simulink model "dualConversionSuperheterodyneKuBandReceiver"  (R2021b)
settings: Solver=VariableStepAuto  StartTime=0.0  StopTime=10.0  RelTol=1e-3
undefined symbols (not defined in the file): fdesignblkfcn, gcbh
libraries: dsparch4 x6, dspsrcs4 x4
settings Model: Creator=Zireael  LastModifiedBy=Zireael

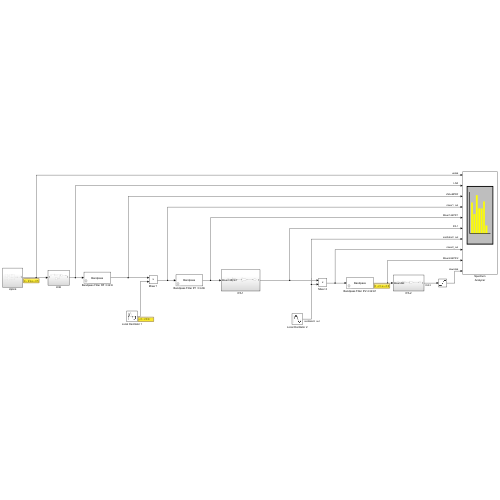
[thumbnail: Simulink's stored preview of the top-level diagram]
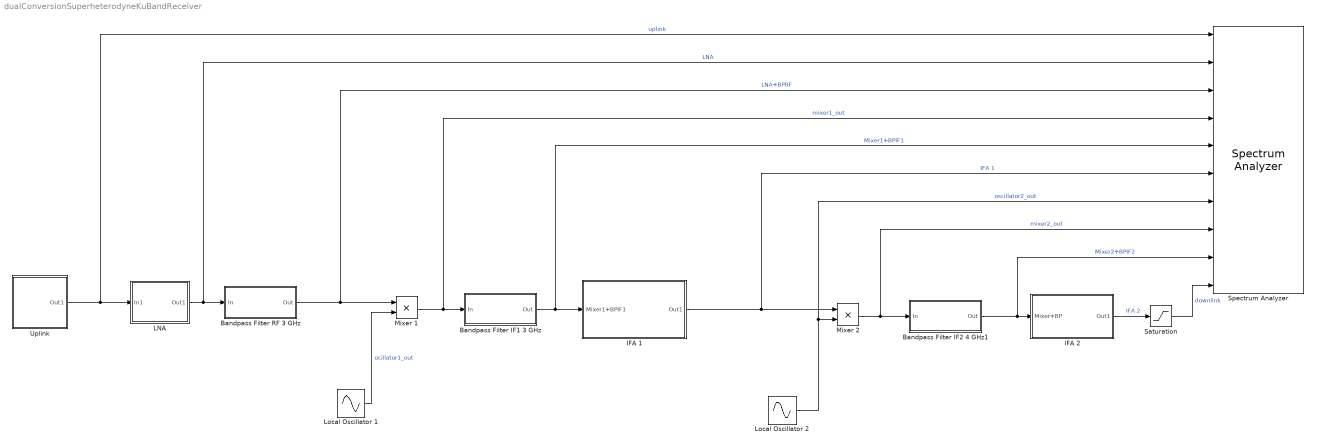
== system dualConversionSuperheterodyneKuBandReceiver ==
  Bandpass Filter IF1 3 GHz : Subsystem  DialogController=fdesignblkfcn  InitFcn=fdesignblkfcn(gcbh, {'InitFcn'});  mask(Bandpass Filter){}
      mask help: Design a bandpass filter
      settings: CopyFcn=fdesignblkfcn(gcbh, {'CopyFcn'});
      mask Help: helpview(mapfilelocation('dsp'), 'dspbandpassfilter');
      mask Display: disp('Bandpass');
  Bandpass Filter IF2 4 GHz1 : Subsystem  DialogController=fdesignblkfcn  InitFcn=fdesignblkfcn(gcbh, {'InitFcn'});  mask(Bandpass Filter){}
      mask help: Design a bandpass filter
      settings: CopyFcn=fdesignblkfcn(gcbh, {'CopyFcn'});
      mask Help: helpview(mapfilelocation('dsp'), 'dspbandpassfilter');
      mask Display: disp('Bandpass');
  Bandpass Filter RF 3 GHz : Subsystem  DialogController=fdesignblkfcn  InitFcn=fdesignblkfcn(gcbh, {'InitFcn'});  mask(Bandpass Filter){}
      mask help: Design a bandpass filter
      settings: CopyFcn=fdesignblkfcn(gcbh, {'CopyFcn'});
      mask Help: helpview(mapfilelocation('dsp'), 'dspbandpassfilter');
      mask Display: disp('Bandpass');
  IFA 1 : Subsystem
  IFA 2 : Subsystem
  LNA : Subsystem
  Local Oscillator 1 : Sin  Frequency=2*pi*2225e6  SampleTime=1/(50e9)
  Local Oscillator 2 : Sin  Frequency=2*pi*2225e6  SampleTime=1/(50e9)
  Mixer 1 : Product
  Mixer 2 : Product
  Saturation : Saturate  UpperLimit=0.9e4  LowerLimit=-0.9e4
  Spectrum Analyzer : SpectrumAnalyzer  NumInputPorts=10
  Uplink : Subsystem
  wires:
  Local Oscillator 1/1 -> Mixer 1/2  "ocillator1_out"
  Uplink/1(Out1) -> Spectrum Analyzer/1, LNA/1(In1)  "uplink"
  Bandpass Filter RF 3 GHz/1(Out) -> Spectrum Analyzer/3, Mixer 1/1  "LNA+BPRF"
  LNA/1(Out1) -> Spectrum Analyzer/2, Bandpass Filter RF 3 GHz/1(In)  "LNA"
  Mixer 1/1 -> Spectrum Analyzer/4, Bandpass Filter IF1 3 GHz/1(In)  "mixer1_out"
  Bandpass Filter IF1 3 GHz/1(Out) -> Spectrum Analyzer/5, IFA 1/1(Mixer1+BPIF1)  "Mixer1+BPIF1"
  Local Oscillator 2/1 -> Mixer 2/2, Spectrum Analyzer/7  "oscillator2_out"
  Mixer 2/1 -> Spectrum Analyzer/8, Bandpass Filter IF2 4 GHz1/1(In)  "mixer2_out"
  Bandpass Filter IF2 4 GHz1/1(Out) -> Spectrum Analyzer/9, IFA 2/1(Mixer+BP)  "Mixer2+BPIF2"
  IFA 1/1(Out1) -> Spectrum Analyzer/6, Mixer 2/1  "IFA 1"
  IFA 2/1(Out1) -> Saturation/1  "IFA 2"
  Saturation/1 -> Spectrum Analyzer/10  "downlink"

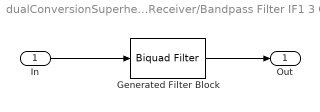
== system dualConversionSuperheterodyneKuBandReceiver/Bandpass Filter IF1 3 GHz ==
  In : Inport
  Generated Filter Block : dsparch4/Biquad Filter  Tag=BlockMethodSubSystem  FilterSource=Dialog parameters  CoeffSource=Specify via dialog  FilterObject=BQF  IIRFiltStruct=Direct form II  BiQuadCoeffs=[0.0449395006068324179 0 -0.0449395006068324179 1 0.405266255527262198 0.993681559777048418;0.0151701499365588764 0 -0.0151701499365588764 1 0.317251182402427279 0.993629226472784288;0.0102846537000260332 0 -0.0102846537000260332 1 0.370702484346910832 0.991152828113709083;0.0156527649221751067 0 -0.0156527649221751067 1 0.351249848252692232 0.991136685128483963;0.0620781828063547217 0 -0.0620781828063547217 1 0.423582164672003603 0.998601688644412899;0.00934586574907354285 0 -0.00934586574907354285 1 0.300377452446864479 0.998585448434978429;0.0223874419851657382 0 -0.0223874419851657382 1 0.389303276704848988 0.992030706822551345;0.0130129978737727608 0 -0.0130129978737727608 1 0.332830940728660596 0.991988419043733027;0.059531840912397431 0 -0.059531840912397431 1 0.417068161267263871 0.995944293101420075;0.511470005384135895 0 -0.511470005384135895 1 0.306057042862860063 0.995901877379559486]  ScaleValues=[0.00618861187356475363;1;1;1;1;1;1;1;1;1;1]  IC=0  ICnum=0  ICden=0  a0Flag=Warning  optimizeScaleValues=off  ScaleValueMode=Specify via input port (g)  InputProcessing=Columns as channels (frame based)  roundingMode=Floor  overflowMode=off  scaleValueFracLength=14  denProdOutputFracLength=30  denAccumFracLength=30  secondMemoryFracLength=15
  Out : Outport  VectorParamsAs1DForOutWhenUnconnected=off
  wires:
  In/1 -> Generated Filter Block/1
  Generated Filter Block/1 -> Out/1

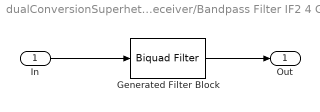
== system dualConversionSuperheterodyneKuBandReceiver/Bandpass Filter IF2 4 GHz1 ==
  In : Inport
  Generated Filter Block : dsparch4/Biquad Filter  Tag=BlockMethodSubSystem  FilterSource=Dialog parameters  CoeffSource=Specify via dialog  FilterObject=BQF  IIRFiltStruct=Direct form II  BiQuadCoeffs=[0.0449395006068324179 0 -0.0449395006068324179 1 0.405266255527262198 0.993681559777048418;0.0151701499365588764 0 -0.0151701499365588764 1 0.317251182402427279 0.993629226472784288;0.0102846537000260332 0 -0.0102846537000260332 1 0.370702484346910832 0.991152828113709083;0.0156527649221751067 0 -0.0156527649221751067 1 0.351249848252692232 0.991136685128483963;0.0620781828063547217 0 -0.0620781828063547217 1 0.423582164672003603 0.998601688644412899;0.00934586574907354285 0 -0.00934586574907354285 1 0.300377452446864479 0.998585448434978429;0.0223874419851657382 0 -0.0223874419851657382 1 0.389303276704848988 0.992030706822551345;0.0130129978737727608 0 -0.0130129978737727608 1 0.332830940728660596 0.991988419043733027;0.059531840912397431 0 -0.059531840912397431 1 0.417068161267263871 0.995944293101420075;0.511470005384135895 0 -0.511470005384135895 1 0.306057042862860063 0.995901877379559486]  ScaleValues=[0.00618861187356475363;1;1;1;1;1;1;1;1;1;1]  IC=0  ICnum=0  ICden=0  a0Flag=Warning  optimizeScaleValues=off  ScaleValueMode=Specify via input port (g)  InputProcessing=Columns as channels (frame based)  roundingMode=Floor  overflowMode=off  scaleValueFracLength=14  denProdOutputFracLength=30  denAccumFracLength=30  secondMemoryFracLength=15
  Out : Outport  VectorParamsAs1DForOutWhenUnconnected=off
  wires:
  In/1 -> Generated Filter Block/1
  Generated Filter Block/1 -> Out/1

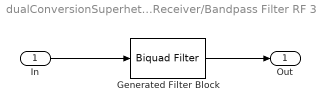
== system dualConversionSuperheterodyneKuBandReceiver/Bandpass Filter RF 3 GHz ==
  In : Inport
  Generated Filter Block : dsparch4/Biquad Filter  Tag=BlockMethodSubSystem  FilterSource=Dialog parameters  CoeffSource=Specify via dialog  FilterObject=BQF  IIRFiltStruct=Direct form II  BiQuadCoeffs=[0.0449015005721064217 0 -0.0449015005721064217 1 0.460304770997229384 0.993685734471094873;0.0151718610592496122 0 -0.0151718610592496122 1 0.372780342872187143 0.993625052016134158;0.010292301404864557 0 -0.010292301404864557 1 0.425888978774519256 0.991154115861604401;0.0155960047074426896 0 -0.0155960047074426896 1 0.406544551045089853 0.991135397403234641;0.0623098100146096748 0 -0.0623098100146096748 1 0.478631344122104563 0.998602984094145718;0.0093415546403119807 0 -0.0093415546403119807 1 0.356116647279347776 0.998584153007991748;0.0223945390284251249 0 -0.0223945390284251249 1 0.444400611296275394 0.992034080197356283;0.0130197808043754238 0 -0.0130197808043754238 1 0.388242637402923141 0.991985045824199996;0.0594862648562931723 0 -0.0594862648562931723 1 0.472088444940327034 0.995947676595487108;0.514535971971806561 0 -0.514535971971806561 1 0.36169744229138806 0.995898494041079996]  ScaleValues=[0.00615350492122296311;1;1;1;1;1;1;1;1;1;1]  IC=0  ICnum=0  ICden=0  a0Flag=Warning  optimizeScaleValues=off  ScaleValueMode=Specify via input port (g)  InputProcessing=Columns as channels (frame based)  roundingMode=Floor  overflowMode=off  scaleValueFracLength=14  denProdOutputFracLength=30  denAccumFracLength=30  secondMemoryFracLength=15
  Out : Outport  VectorParamsAs1DForOutWhenUnconnected=off
  wires:
  In/1 -> Generated Filter Block/1
  Generated Filter Block/1 -> Out/1

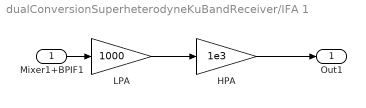
== system dualConversionSuperheterodyneKuBandReceiver/IFA 1 ==
  Mixer1+BPIF1 : Inport
  HPA : Gain  Gain=1e3
  LPA : Gain  Gain=1000
  Out1 : Outport
  wires:
  Mixer1+BPIF1/1 -> LPA/1
  LPA/1 -> HPA/1
  HPA/1 -> Out1/1

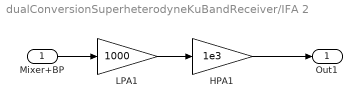
== system dualConversionSuperheterodyneKuBandReceiver/IFA 2 ==
  Mixer+BP : Inport
  HPA1 : Gain  Gain=1e3
  LPA1 : Gain  Gain=1000
  Out1 : Outport
  wires:
  LPA1/1 -> HPA1/1
  HPA1/1 -> Out1/1
  Mixer+BP/1 -> LPA1/1

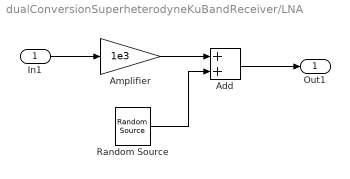
== system dualConversionSuperheterodyneKuBandReceiver/LNA ==
  In1 : Inport
  Add : Sum
  Amplifier : Gain  Gain=1e3
  Random Source : dspsrcs4/Random Source  SrcType=Gaussian  NormMethod=Ziggurat  CltLength=12  MinVal=0  MaxVal=1  MeanVal=0  VarVal=1e-3  RepMode=Not repeatable  rawSeed=1  IsInherit=off  SampMode=Discrete  SampTime=1/(50e9)  SampFrame=1  DataType=Double  OutComplex=Real  OutputFrames=off
  Out1 : Outport
  wires:
  Random Source/1 -> Add/2
  Amplifier/1 -> Add/1
  Add/1 -> Out1/1
  In1/1 -> Amplifier/1

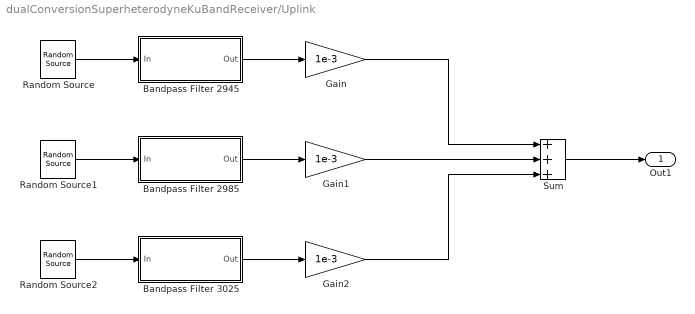
== system dualConversionSuperheterodyneKuBandReceiver/Uplink ==
  Bandpass Filter 2945 : Subsystem  DialogController=fdesignblkfcn  InitFcn=fdesignblkfcn(gcbh, {'InitFcn'});  mask(Bandpass Filter){}
      mask help: Design a bandpass filter
      settings: CopyFcn=fdesignblkfcn(gcbh, {'CopyFcn'});
      mask Help: helpview(mapfilelocation('dsp'), 'dspbandpassfilter');
      mask Display: disp('Bandpass');
  Bandpass Filter 2985 : Subsystem  DialogController=fdesignblkfcn  InitFcn=fdesignblkfcn(gcbh, {'InitFcn'});  mask(Bandpass Filter){}
      mask help: Design a bandpass filter
      settings: CopyFcn=fdesignblkfcn(gcbh, {'CopyFcn'});
      mask Help: helpview(mapfilelocation('dsp'), 'dspbandpassfilter');
      mask Display: disp('Bandpass');
  Bandpass Filter 3025 : Subsystem  DialogController=fdesignblkfcn  InitFcn=fdesignblkfcn(gcbh, {'InitFcn'});  mask(Bandpass Filter){}
      mask help: Design a bandpass filter
      settings: CopyFcn=fdesignblkfcn(gcbh, {'CopyFcn'});
      mask Help: helpview(mapfilelocation('dsp'), 'dspbandpassfilter');
      mask Display: disp('Bandpass');
  Gain : Gain  Gain=1e-3
  Gain1 : Gain  Gain=1e-3
  Gain2 : Gain  Gain=1e-3
  Random Source : dspsrcs4/Random Source  SrcType=Gaussian  NormMethod=Ziggurat  CltLength=12  MinVal=0  MaxVal=1  MeanVal=0  VarVal=1  RepMode=Not repeatable  rawSeed=1  IsInherit=off  SampMode=Discrete  SampTime=1/(50e9)  SampFrame=1  DataType=Double  OutComplex=Real  OutputFrames=off
  Random Source1 : dspsrcs4/Random Source  SrcType=Gaussian  NormMethod=Ziggurat  CltLength=12  MinVal=0  MaxVal=1  MeanVal=0  VarVal=1  RepMode=Not repeatable  rawSeed=1  IsInherit=off  SampMode=Discrete  SampTime=1/(50e9)  SampFrame=1  DataType=Double  OutComplex=Real  OutputFrames=off
  Random Source2 : dspsrcs4/Random Source  SrcType=Gaussian  NormMethod=Ziggurat  CltLength=12  MinVal=0  MaxVal=1  MeanVal=0  VarVal=1  RepMode=Not repeatable  rawSeed=1  IsInherit=off  SampMode=Discrete  SampTime=1/(50e9)  SampFrame=1  DataType=Double  OutComplex=Real  OutputFrames=off
  Sum : Sum  Inputs=+++
  Out1 : Outport
  wires:
  Random Source/1 -> Bandpass Filter 2945/1(In)
  Bandpass Filter 2945/1(Out) -> Gain/1
  Bandpass Filter 2985/1(Out) -> Gain1/1
  Random Source1/1 -> Bandpass Filter 2985/1(In)
  Random Source2/1 -> Bandpass Filter 3025/1(In)
  Bandpass Filter 3025/1(Out) -> Gain2/1
  Sum/1 -> Out1/1
  Gain/1 -> Sum/1
  Gain1/1 -> Sum/2
  Gain2/1 -> Sum/3

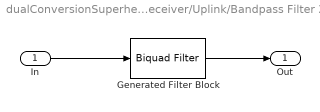
== system dualConversionSuperheterodyneKuBandReceiver/Uplink/Bandpass Filter 2945 ==
  In : Inport
  Generated Filter Block : dsparch4/Biquad Filter  Tag=BlockMethodSubSystem  FilterSource=Dialog parameters  CoeffSource=Specify via dialog  FilterObject=BQF  IIRFiltStruct=Direct form II  BiQuadCoeffs=[0.00405053939434224779 0 -0.00405053939434224779 1 0.365006670153093293 0.999784442609443325;0.00115477981683422839 0 -0.00115477981683422839 1 0.357265743093537813 0.999784286808510614;0.00106672134041485242 0 -0.00106672134041485242 1 0.362029406066514792 0.999578232245606157;0.000673674460618607683 0 -0.000673674460618607683 1 0.360171179090651716 0.999578159086874751;0.00222185254217866033 0 -0.00222185254217866033 1 0.363739676780378884 0.999651202827206098;0.000967942063617497836 0 -0.000967942063617497836 1 0.358486119058677777 0.999651031751173536;0.00412407482795272735 0 -0.00412407482795272735 1 0.365611667239622518 0.999954934864948464;0.000214662508465945359 0 -0.000214662508465945359 1 0.356721453146472411 0.999954897454661706;0.00341656386874102363 0 -0.00341656386874102363 1 0.364444571914590509 0.999711523336087371;0.00173805995246988196 0 -0.00173805995246988196 1 0.357802237861854 0.999711344430960436;0.000520610924197030013 0 -0.000520610924197030013 1 0.361098671752999478 0.999568774242084457;0.00168833692563991446 0 -0.00168833692563991446 1 0.36292273886777765 0.999606115496003311;0.0010404353766466411 0 -0.0010404353766466411 1 0.359287450545718146 0.999605981825039125;0.00401366133462534476 0 -0.00401366133462534476 1 0.365401445992077245 0.999866777555257213;0.507701145002624754 0 -0.507701145002624754 1 0.356900137362369585 0.999866671802023044]  ScaleValues=[0.000350900431951329324;1;1;1;1;1;1;1;1;1;1;1;1;1;1;1]  IC=0  ICnum=0  ICden=0  a0Flag=Warning  optimizeScaleValues=off  ScaleValueMode=Specify via input port (g)  InputProcessing=Columns as channels (frame based)  roundingMode=Floor  overflowMode=off  scaleValueFracLength=14  denProdOutputFracLength=30  denAccumFracLength=30  secondMemoryFracLength=15
  Out : Outport  VectorParamsAs1DForOutWhenUnconnected=off
  wires:
  In/1 -> Generated Filter Block/1
  Generated Filter Block/1 -> Out/1

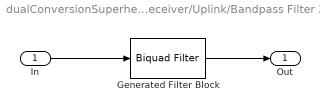
== system dualConversionSuperheterodyneKuBandReceiver/Uplink/Bandpass Filter 2985 ==
  In : Inport
  Generated Filter Block : dsparch4/Biquad Filter  Tag=BlockMethodSubSystem  FilterSource=Dialog parameters  CoeffSource=Specify via dialog  FilterObject=BQF  IIRFiltStruct=Direct form II  BiQuadCoeffs=[0.00403925271348525104 0 -0.00403925271348525104 1 0.374885179221466469 0.999784444816041451;0.00132591425811228749 0 -0.00132591425811228749 1 0.36715149247363893 0.9997842846019106;0.00102874696105771462 0 -0.00102874696105771462 1 0.371909683694259474 0.999578233281725015;0.000735878605933630776 0 -0.000735878605933630776 1 0.37005319440792428 0.999578158050755228;0.00209164582786390768 0 -0.00209164582786390768 1 0.373618711616941546 0.999651205250157937;0.000964620228458040806 0 -0.000964620228458040806 1 0.368370067032101678 0.999651029328230023;0.00433052574112255742 0 -0.00433052574112255742 1 0.375490468694301471 0.999954935394811395;0.00021779640289240363 0 -0.00021779640289240363 1 0.366608571330107491 0.999954896924799219;0.00337757846451481551 0 -0.00337757846451481551 1 0.374323244680184464 0.999711525869927398;0.00169870066657281239 0 -0.00169870066657281239 1 0.3676871229315129 0.999711341897121186;0.000535022730231889403 0 -0.000535022730231889403 1 0.370979773873246821 0.999568774242085234;0.00165541231778167097 0 -0.00165541231778167097 1 0.372802316959541302 0.99960611738931382;0.00111483261478020944 0 -0.00111483261478020944 1 0.369170428209791734 0.999605979931723176;0.00384792957152922622 0 -0.00384792957152922622 1 0.375279998227074252 0.999866779052987709;0.508910309410927519 0 -0.508910309410927519 1 0.366786641786524148 0.999866670304293104]  ScaleValues=[0.000290328198979075257;1;1;1;1;1;1;1;1;1;1;1;1;1;1;1]  IC=0  ICnum=0  ICden=0  a0Flag=Warning  optimizeScaleValues=off  ScaleValueMode=Specify via input port (g)  InputProcessing=Columns as channels (frame based)  roundingMode=Floor  overflowMode=off  scaleValueFracLength=14  denProdOutputFracLength=30  denAccumFracLength=30  secondMemoryFracLength=15
  Out : Outport  VectorParamsAs1DForOutWhenUnconnected=off
  wires:
  In/1 -> Generated Filter Block/1
  Generated Filter Block/1 -> Out/1

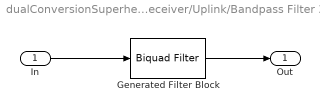
== system dualConversionSuperheterodyneKuBandReceiver/Uplink/Bandpass Filter 3025 ==
  In : Inport
  Generated Filter Block : dsparch4/Biquad Filter  Tag=BlockMethodSubSystem  FilterSource=Dialog parameters  CoeffSource=Specify via dialog  FilterObject=BQF  IIRFiltStruct=Direct form II  BiQuadCoeffs=[0.00412481187045002883 0 -0.00412481187045002883 1 0.385021640166252122 0.999876346309697239;0.000853824778251791993 0 -0.000853824778251791993 1 0.376795167022748678 0.999876245747868264;0.00321596008473088368 0 -0.00321596008473088368 1 0.383206677359378411 0.999724464069084773;0.000767567853297673221 0 -0.000767567853297673221 1 0.378554542219186663 0.999724337372378313;0.00103480614175016552 0 -0.00103480614175016552 1 0.381912904755242255 0.999685738420582393;0.000840361445624580937 0 -0.000840361445624580937 1 0.379834430629378383 0.999685673867775071;0.00298750732208348871 0 -0.00298750732208348871 1 0.38427781219166296 0.999790142265788995;0.000543644444719714208 0 -0.000543644444719714208 1 0.377507228183375232 0.999790001812424944;0.00402463995530418558 0 -0.00402463995530418558 1 0.385365478443618181 0.999974647675154982;0.000134871645340931115 0 -0.000134871645340931115 1 0.376488239997609109 0.999974625425492869;0.00396342849366130689 0 -0.00396342849366130689 1 0.38469603187083512 0.999831167282022815;0.00116920940940745286 0 -0.00116920940940745286 1 0.377104056036845936 0.999831040572199625;0.00289955111711492908 0 -0.00289955111711492908 1 0.38258009039976193 0.999701427502675322;0.000900652680936045338 0 -0.000900652680936045338 1 0.379172854479336074 0.999701326957836867;0.000616486781974766589 0 -0.000616486781974766589 1 0.381221529231434098 0.999677784136744574;0.00105243171093662852 0 -0.00105243171093662852 1 0.380522973494800576 0.999677761893515537;0.00206349250860282185 0 -0.00206349250860282185 1 0.383777259844310992 0.999754280372320725;0.00122769552612205478 0 -0.00122769552612205478 1 0.3779947323582033 0.999754139923923479;0.0038038816740453619 0 -0.0038038816740453619 1 0.385246633364180913 0.999924568338884878;0.508628235300513598 0 -0.508628235300513598 1 0.376588189688731145 0.999924503771082884]  ScaleValues=[0.00017927175844706573;1;1;1;1;1;1;1;1;1;1;1;1;1;1;1;1;1;1;1;1]  IC=0  ICnum=0  ICden=0  a0Flag=Warning  optimizeScaleValues=off  ScaleValueMode=Specify via input port (g)  InputProcessing=Columns as channels (frame based)  roundingMode=Floor  overflowMode=off  scaleValueFracLength=14  denProdOutputFracLength=30  denAccumFracLength=30  secondMemoryFracLength=15
  Out : Outport  VectorParamsAs1DForOutWhenUnconnected=off
  wires:
  Generated Filter Block/1 -> Out/1
  In/1 -> Generated Filter Block/1
